simulink model "MASH20_Bader_Float64"  (R2023b)
settings: Solver=ode45  StartTime=0.0  StopTime=1  MaxStep=Ts/10  EnableMultiTasking=on
PreLoadFcn:
  | s0=sprintf('===========================================================================');disp(s0)
  | s1=sprintf('= Created by Bader Almutair bmutairi@kacst.edu.sa                         =');disp(s1)
  | s2=sprintf('= Date 12/11/2014                                                         =');disp(s2)
  | s3=sprintf('= Refer to the PhD thesis Ch4,P.55                                        =');disp(s3)
  | s4=sprintf('===========================================================================');disp(s4)
values from neighbouring files (symbols this model uses):
  AA = AA_design*(mismatch_lower_limit + rand_range*rand)    [simon_test.m]    (also in testPSD_simulink.m)
  b = b_design*(0.8 + (1.2 - 0.8) * rand)    [D2_parameter_mapping.m]    (also in simon_test.m = b_design*(mismatch_lower_limit + rand_range*rand); testPSD_simulink.m = b_design*(mismatch_lower_limit + rand_range*rand))
  d0 = d0_design*(mismatch_lower_limit + rand_range*rand)    [simon_test.m]    (also in testPSD_simulink.m)
  enoise = 10e-9    (= 1e-08)    [simon_test.m]    (also in testPSD_simulink.m)
  epsilon = 8.854e-12    [population_score_c2d.m]    (also in simon_test.m; testPSD_c2d.m; testPSD_simulink.m)
  Finput = F_resolution*128    (= 260.4140625)    [new_generation_coeff.m]    (also in simon_test.m; testPSD_simulink.m)
  k = k_design*(0.8 + (1.2 - 0.8) * rand)    [D2_parameter_mapping.m]    (also in log2_linear_taylor.m = floor(log2(x)); population_score.m = floor(log2(real(Y3).^2 + imag(Y3).^2)); population_score_c2d.m = floor(log2(Y3)); simon_test.m = k_design*(mismatch_lower_limit + rand_range*rand))
  Kfb = Kfb_design*(0.8 + (1.2 - 0.8) * rand)    [D2_parameter_mapping.m]    (also in simon_test.m = 0.5*epsilon*AA*(Vfeedback^2)/(d0^2); testPSD_simulink.m = 0.5*epsilon*AA*(Vfeedback^2)/(d0^2))
  Kpo = Kpo_design*(0.8 + (1.2 - 0.8) * rand)    [D2_parameter_mapping.m]    (also in simon_test.m = Kpo_design*(mismatch_lower_limit + rand_range*rand); testPSD_simulink.m = Kpo_design*(mismatch_lower_limit + rand_range*rand))
  Lfactor = Vfeedback/d0    [simon_test.m]    (also in testPSD_simulink.m)
  m = m_design*(0.8 + (1.2 - 0.8) * rand)    [D2_parameter_mapping.m]    (also in simon_test.m = m_design*(mismatch_lower_limit + rand_range*rand); testPSD_simulink.m = m_design*(mismatch_lower_limit + rand_range*rand))
  pole = alpha*zero    [simon_test.m]    (also in testPSD_c2d.m; testPSD_simulink.m)
  Ts = 1/Fs    (= 7.50007500075e-06)    [new_generation_coeff.m]    (also in simon_test.m; simple_fft_test.m = 1/F; testPSD_c2d.m; testPSD_simulink.m)
  Vfeedback = Vfeedback_design*(mismatch_lower_limit + rand_range*rand)    [simon_test.m]    (also in testPSD_simulink.m)
  x = linspace(min(a4), max(a4), 100)    [D2_parameter_mapping.m]    (also in log2_linear_taylor.m = 1e-10; simon_test.m = 0.9; testPSD_simulink.m = 0.9)
  zero = WL/sqrt(alpha)    [simon_test.m]    (also in testPSD_c2d.m; testPSD_simulink.m)
undefined symbols (not defined in the file or in its folder): D1den, D1num, D2den, D2num, Digital_Compv2_den, Digital_Compv2_num
libraries: simulink_extras x2, dspfdesign x2, dspsigops x1
settings Model: Creator=Administrator  LastModifiedBy=Simon
settings SolverCC: AlgebraicLoopSolver=TrustRegion
settings DataIOCC: LimitDataPoints=on  SaveFormat=Array  SignalLoggingSaveFormat=ModelDataLogs  ReturnWorkspaceOutputs=off
settings OptimizationCC: ReuseModelBlockBuffer=off  ExpressionDepthLimit=2147483647  LifeSpan=inf
settings DebuggingCC: UnderspecifiedInitializationDetection=Classic  MergeDetectMultiDrivingBlocksExec=none  SolverPrmCheckMsg=warning  FcnCallInpInsideContextMsg=warning  UnconnectedInputMsg=warning  UnconnectedOutputMsg=warning  UnconnectedLineMsg=warning  StateNameClashWarn=warning  SFUnexpectedBacktrackingDiag=warning  SFNoUnconditionalDefaultTransitionDiag=warning  SFExecutionAtInitializationDiag=none  ArithmeticOperatorsInVariantConditions=warning
settings HardwareCC: ProdBitPerPointer=32  ProdBitPerSizeT=32  ProdBitPerPtrDiffT=32  ProdLargestAtomicFloat=None  ProdIntDivRoundTo=Undefined  ProdEndianess=Unspecified  ProdWordSize=32  ProdHWDeviceType=32-bit Generic
settings ModelReferenceCC: PropagateSignalLabelsOutOfModel=off
settings SFSimCC: SimUseLocalCustomCode=off  CustomCodeUndefinedFunction=UseInterfaceOnly
settings RTWCC: RTWUseLocalCustomCode=off
settings CodeAppCC: StateflowObjectComments=on
settings GRTTargetCC: TargetLangStandard=C89/C90 (ANSI)  CombineOutputUpdateFcns=off  GRTInterface=on
settings ConfigComp: CovMetricSettings=dw  CovSaveCumulativeToWorkspaceVar=on  CovSaveSingleToWorkspaceVar=on  CovExternalEMLEnable=off

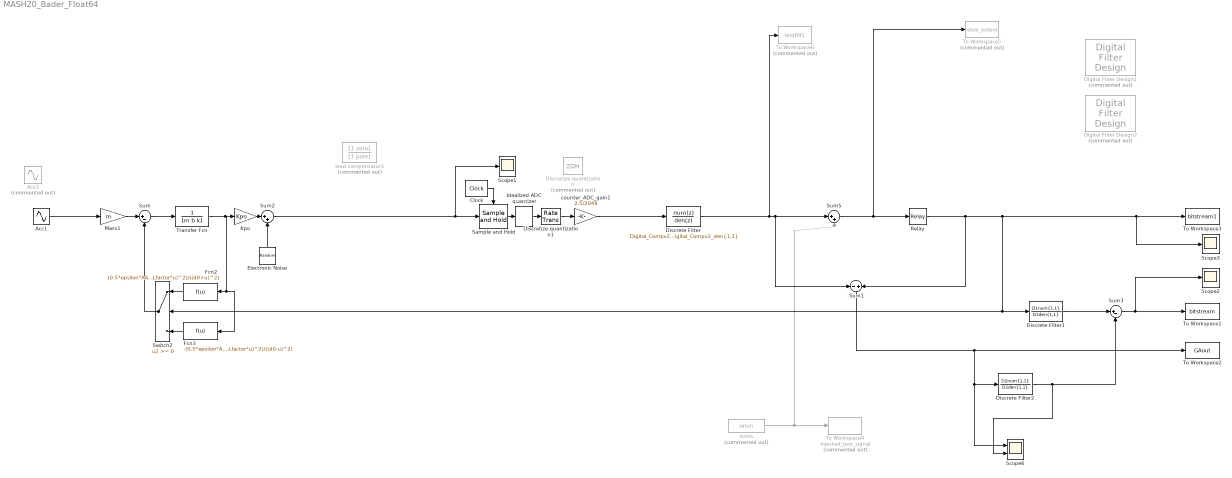
== system MASH20_Bader_Float64 ==
  Acc1 : Sin  Amplitude=(Kfb/m)*x  Frequency=Finput*2*pi  SampleTime=0
  Acc2 : Sin  Commented=on  Amplitude=(Kfb/m)*x  Frequency=Finput*2*pi  SampleTime=0
  Clock : simulink_extras/Flip Flops/Clock  period=Ts
  Digital Filter Design1 : dspfdesign/Digital Filter Design  Commented=on  mwdsp_browser_bugfix_var=off
  Digital Filter Design2 : dspfdesign/Digital Filter Design  Commented=on  mwdsp_browser_bugfix_var=off
  Discrete Filter : DiscreteFilter  Numerator=Digital_Compv2_num{1,1}  Denominator=Digital_Compv2_den{1,1}  FilterStructure=Direct form II transposed
  Discrete Filter1 : DiscreteFilter  Numerator=D1num{1,1}  Denominator=D1den{1,1}  FilterStructure=Direct form II transposed
  Discrete Filter2 : DiscreteFilter  Numerator=D2num{1,1}  Denominator=D2den{1,1}
  Discretize quantization : ZeroOrderHold  Commented=on  SampleTime=Ts
  Discretize quantization1 : RateTransition  OutPortSampleTime=Ts
  Electronic Noise : RandomNumber  Variance=(enoise*sqrt(5/Ts))^2  Seed=432  SampleTime=Ts
  Fcn2 : Fcn  Expr=(0.5*epsilon*AA*(Vfeedback+Lfactor*u)^2)/((d0+u)^2)
  Fcn3 : Fcn  Expr=-(0.5*epsilon*AA*(Vfeedback-Lfactor*u)^2)/((d0-u)^2)
  Idealized ADC quantizer : simulink_extras/Additional Discrete/Idealized ADC quantizer  NumberOfConverterBits=12  Vmin=-2.5  Vmax=2.5  OutputDataType=double  OutputNegativeValues=on
  Kpo : Gain  Gain=Kpo
  Mass1 : Gain  Gain=m
  Relay : Relay  OffOutputValue=-1  OutDataTypeStr=Inherit: Inherit via back propagation
  Sample and Hold : dspsigops/Sample and Hold  trig=Rising edge  initCond=0  latchinput=off
  Scope1 : Scope
  Scope2 : Scope
  Scope3 : Scope
  Scope6 : Scope  NumInputPorts=2
  Sum : Sum  Inputs=|+-
  Sum1 : Sum  Inputs=-+  InputSameDT=on
  Sum2 : Sum  Inputs=|++
  Sum3 : Sum  Inputs=|+-
  Sum5 : Sum  Inputs=|++  InputSameDT=on
  Switch2 : Switch  SaturateOnIntegerOverflow=off  InputSameDT=off
  To Workspace1 : ToWorkspace  VariableName=bitstream  SampleTime=Ts
  To Workspace2 : ToWorkspace  VariableName=GAout  SampleTime=Ts
  To Workspace3 : ToWorkspace  VariableName=bitstream1  SampleTime=Ts
  To Workspace4 : ToWorkspace  Commented=on  VariableName=injected_test_signal  SampleTime=Ts
  To Workspace5 : ToWorkspace  Commented=on  VariableName=ideal_output  SampleTime=Ts
  To Workspace6 : ToWorkspace  Commented=on  VariableName=test691  SampleTime=Ts
  Transfer Fcn : TransferFcn  Denominator=[m b k]
  counter_ADC_gain1 : Gain  Gain=2.5/2048  OutDataTypeStr=double
  lead compensator3 : TransferFcn  Commented=on  Numerator=[1 zero]  Denominator=[1 pole]
  simin : FromWorkspace  Commented=on  VariableName=simin  Interpolate=off  OutputAfterFinalValue=Holding final value
  wires:
  Transfer Fcn/1 -> Fcn3/1, Fcn2/1, Kpo/1
  Sum/1 -> Transfer Fcn/1
  Mass1/1 -> Sum/1
  Fcn2/1 -> Switch2/1
  Fcn3/1 -> Switch2/3
  Switch2/1 -> Sum/2
  Kpo/1 -> Sum2/1
  Electronic Noise/1 -> Sum2/2
  Sum3/1 -> Scope2/1, To Workspace1/1
  simin/1 -> To Workspace4/1, Sum5/2
  Sample and Hold/1 -> Idealized ADC quantizer/1
  Clock/1 -> Sample and Hold/Trigger
  Acc1/1 -> Mass1/1
  Sum2/1 -> Scope1/1, Sample and Hold/1
  counter_ADC_gain1/1 -> Discrete Filter/1
  Idealized ADC quantizer/1 -> Discretize quantization1/1
  Discrete Filter2/1 -> Sum3/2, Scope6/2
  Sum1/1 -> Discrete Filter2/1, Scope6/1, To Workspace2/1
  Sum5/1 -> Relay/1, To Workspace5/1
  Discrete Filter/1 -> Sum1/1, Sum5/1, To Workspace6/1
  Relay/1 -> Sum1/2, To Workspace3/1, Scope3/1, Discrete Filter1/1, Switch2/2
  Discretize quantization1/1 -> counter_ADC_gain1/1
  Discrete Filter1/1 -> Sum3/1
